simulink model "elec_auto_ev_simulink"  (R2017b)
settings: Solver=FixedStepAuto  StartTime=0.0  StopTime=200  RelTol=1e-3  AbsTol=1e-3
PreLoadFcn:
  | % Simulation parameters
  | dt = 0.01;
  | 
  | % Battery cell parameters
  | ssc_lithium_cell_1RC_ini
  | 
  | % Motor parameters
  | max_torque = 220;
  | max_power = 50e3;
  | 
  | % Vehicle parameters
  | vehicle_mass = 1000;
  | wheel_radius = 0.25;
  | area = 5;
  | drag_coefficient = 0.25;
  | air_density = 1.225;
  | gravity = 9.81;
  | rolling_res_ratio = 0.015;
  | 
  | % Differential drive parameters
  | gear_ratio = 6;
  | 
  | % Simplified braking system parameters
  | force_max_pedal = 500;
  | braking_torque_to_pedal_force_ratio = -4;
  | 
  | % Vehicle controller parameters
  | hill_hold_max_speed = 0.5;
  | 
  | % Water properties for cooling circuit
  | load WaterProperties
undefined symbols (not defined in the file): C1_LUT, Capacity_LUT, cell_Cp_heat, cell_mass, DiscIntNeverNeededParam, Em_LUT, Qe_init, R0_LUT, R1_LUT, sigbuilder_block, SOC_LUT, T_init, Temperature_LUT
libraries: fl_lib x93, nesl_utility x12, LiBatteryElements_lib x4, elec_lib x2, simulink x2, simulink_extras x1
(part 1 of 2)
CloseFcn:
  | try,close(h1_elec_auto_ev),end
  | clear h1_elec_auto_ev
  | try,close(h2_elec_auto_ev),end
  | clear h2_elec_auto_ev
  | 
  | clear simlog_elec_auto_ev
  | clear logsout_elec_auto_ev
Description:
  | Electric Vehicle Configured for HIL
  | 
  | Copyright 2008-2017 The MathWorks, Inc.
settings Model: Creator=MathWorks  LastModifiedBy=Sivakumar
settings SolverCC: InitialStep=1e-3
settings DataIOCC: MaxDataPoints=30000  SaveFormat=Array  SignalLoggingName=logsout_elec_auto_ev
settings OptimizationCC: BlockReduction=off  BooleanDataType=off  LifeSpan=inf
settings DebuggingCC: SaveWithParameterizedLinksMsg=none  UnderspecifiedInitializationDetection=Classic  MergeDetectMultiDrivingBlocksExec=none  SignalResolutionControl=TryResolveAllWithWarning  AllowSymbolicDim=off  SFUnexpectedBacktrackingDiag=warning  SFNoUnconditionalDefaultTransitionDiag=warning  SFExecutionAtInitializationDiag=none
settings HardwareCC: ProdBitPerPointer=32  ProdBitPerSizeT=32  ProdBitPerPtrDiffT=32  ProdLargestAtomicFloat=None  ProdIntDivRoundTo=Undefined  ProdEndianess=Unspecified  ProdWordSize=32  ProdHWDeviceType=32-bit Generic  TargetUnknown=on
settings ModelReferenceCC: PropagateSignalLabelsOutOfModel=off
settings CodeAppCC: StateflowObjectComments=on
settings GRTTargetCC: TargetLangStandard=C89/C90 (ANSI)  GeneratePreprocessorConditionals=Disable all
settings ConfigComp: CovMetricSettings=dw  CovHtmlReporting=on  CovSaveCumulativeToWorkspaceVar=on  CovSaveSingleToWorkspaceVar=on  CovExternalEMLEnable=off  CovSFcnEnable=off
settings SimscapeCC: SimscapeLogType=all  SimscapeLogSimulationStatistics=on  SimscapeLogName=simlog_elec_auto_ev  SimscapeLogDataHistory=30000

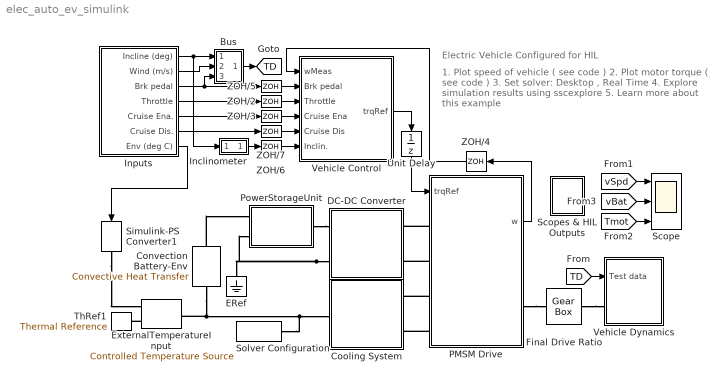
== system elec_auto_ev_simulink ==
  note: Electric Vehicle Configured for HIL
  note: 1. Plot speed of vehicle ( see code )
      | 2. Plot motor torque ( see code )
      | 3. Set solver: Desktop , Real Time
      | 4. Explore simulation results using sscexplore
      | 5. Learn more about this example
  ExternalTemperatureInput : fl_lib/Thermal/Thermal Sources/Controlled Temperature Source
      settings: SourceProductName=Foundation Library
  PowerStorageUnit : Subsystem  mask(Lithium cell (one RC-branch equivalent circuit)){Nseries=50, Nparallel=10, Qe_init=Qe_init, T_init=T_init, Capacity_LUT=Capacity_LUT, Em_LUT=Em_LUT, R0_LUT=R0_LUT, R1_LUT=R1_LUT, C1_LUT=C1_LUT, cell_mass=cell_mass, cell_Cp_heat=cell_Cp_heat, SOC_LUT=SOC_LUT, Temperature_LUT=Temperature_LUT}
      mask prompts: Nseries "Number of series-connected cells"; Nparallel "Number of parallel sets of series-connected cells"; Qe_init "Initial cell charge deficit (A*hr)"; T_init "Initial cell temperature (K)"; Capacity_LUT "Capacity (A*hr, 1xN table)"; Em_LUT "Em open-circuit voltage, Em (volts, MxN table)"; R0_LUT "R0 terminal resistance (ohms, MxN table)"; R1_LUT "R1 cell resistance (ohms, MxN table)"; C1_LUT "C1 capacitance (farads, MxN table)"; cell_mass "Cell mass (kg)"; cell_Cp_heat "Cell specific heat (J/kg/K)"; SOC_LUT "SOC table breakpoints (Mx1 array)"; Temperature_LUT "Temperature table breakpoints (K, 1xN array)"
      mask DialogControl ParameterTabVar0 Prompt: Main
      mask DialogControl ParameterTabVar01 Prompt: Electrical (per cell)
      mask DialogControl ParameterTabVar012 Prompt: Thermal (per cell)
      mask DialogControl ParameterTabVar0123 Prompt: Table Breakpoints
      mask Display:
      | % Battery icon
      | plot([1.8 1.3],[0 0])
      | plot([-0.6 -1.6 -1.6 -2.2],[0 0 -0.9 -0.9])
      | patch([1 1 -1 -1]*0.15+0.7,[-1 1 1 -1]*0.4,[0;0;0]);
      | patch([1 1 -1 -1]*0.15-0.6,[-1 1 1 -1]*0.4,[0;0;0]);
      | patch([1 1 -1 -1]*0.15+1.3,[-1 1 1 -1]*0.8,[0;0;0]);
      | patch([1 1 -1 -1]*0.15-0.0,[-1 1 1 -1]*0.8,[0;0;0]);
      | % Thermal port
      | plot([-1.6,-1.3],[1.2,1.2])
      | plot([-1.6,-1.3],[0.5,0.5])
      | plot([-1.6,-2.5],[0.8,0.8])
      | plot(0.2*sin(0:2*pi/50:2*pi)-1.6,0.35*cos(0:2*pi/50:2*pi)+0.85)
      | plot(0.2*sin(0:2*pi/50:pi)-1.3,0.35*cos(0:2*pi/50:pi)+0.85)
      | 
      | % Plot points to set plot range
      | color('white');plot(2.5,1.5);plot(-2.5,-1.5)
  Bus : Subsystem
  Convection Battery-Env : fl_lib/Thermal/Thermal Elements/Convective Heat Transfer  area=cell_area m^2  heat_tr_coeff=h_conv W/(m^2 * K)  T_specify=off  T_priority=High  T=0 K  T_nominal_specify=off  T_nominal_unit=K  T_nominal_value=1  Q_specify=off  Q_priority=High  Q=0 J/s  Q_nominal_specify=off  Q_nominal_unit=J/s  Q_nominal_value=1
      settings: SourceProductName=Foundation Library
  Cooling System : Subsystem  Tag=PublishSubsystem
  DC-DC Converter : Subsystem
  ERef : fl_lib/Electrical/Electrical Elements/Electrical Reference
      settings: SourceProductName=Foundation Library
  Final Drive Ratio : fl_lib/Mechanical/Mechanisms/Gear Box  ratio=gear_ratio  t_in_specify=off  t_in_priority=High  t_in=0 N*m  t_in_nominal_specify=off  t_in_nominal_unit=N*m  t_in_nominal_value=1  t_out_specify=off  t_out_priority=High  t_out=0 N*m  t_out_nominal_specify=off  t_out_nominal_unit=N*m  t_out_nominal_value=1
      settings: SourceProductName=Foundation Library
  Inclinometer : Subsystem
  Inputs : Subsystem  Tag=STV Subsys  LoadFcn=sigbuilder_block('load');  StartFcn=sigbuilder_block('start');  StopFcn=sigbuilder_block('stop');  ClipboardFcn=sigbuilder_block('clipboard');  mask(Sigbuilder block){tuvar=[0:10]}
      mask help: Simulink:masks:SigbuilderBlock_MD
      mask init:
      | if ~strcmp(get_param(bdroot(gcbh),'SimulationStatus'),'stopped') tuvar = sigbuilder_block('maskInit'); end
      settings: CopyFcn=sigbuilder_block('copy');  DeleteFcn=sigbuilder_block('delete');  ModelCloseFcn=sigbuilder_block('modelClose');  PreSaveFcn=sigbuilder_block('preSave');  PauseFcn=sigbuilder_block('pause');  ContinueFcn=sigbuilder_block('continue');  NameChangeFcn=sigbuilder_block('namechange');  OpenFcn=sigbuilder_block('open',[410.4 81.6 632.4 557.4 ]);  CloseFcn=sigbuilder_block('close');
      mask Display: plot(0, 0, 100, 100,[2, 2, 32, 32, 2], [68, 8, 8, 68, 68],[32, 2], [38, 38], [32, 19, 2],[53, 60, 44], [32, 17, 17, 2],[16, 16, 31, 31]);txt = getActiveGroup(gcbh);text(2, 100, txt,'verticalAlignment', 'top');
  PMSM Drive : Subsystem  Tag=PublishSubsystem  VariantControl=Variant1
  Scope : Scope  NumInputPorts=3
  Scopes & HIL Outputs : Subsystem
  Simulink-PS Converter1 : nesl_utility/Simulink-PS Converter  PhysicalDomain=network_engine_domain  SubClassName=ps_input  LeftPortType=input  RightPortType=output  PseudoPeriodic=off  Frequencies=[]  NoiseDistribution=none  NoiseParameters=[]  Unit=degC  AffineConversion=on  FilteringAndDerivatives=zero  SimscapeFilterOrder=1  InputFilterTimeConstant=.001  UdotUserProvided=1
  Solver Configuration : nesl_utility/Solver Configuration  PhysicalDomain=network_engine_domain  SubClassName=solver  LeftPortType=input  RightPortType=generic  Accelerate=off  Tones=[]  Harmonics=[]  SimulateNoise=off  Profile=off  UseLocalSampling=off  EnableSwitchedLinearOptims=on  FrequencyDomain=off  UseCCode=off  RelTol=0.001  AbsTol=1e-06  MinStep=1e-09  ToWorkspace=off  RevertToSquareIcSolve=off  NumHomotopyIterations=100  PhasorMode=off  PhasorModeNumHarmonics=1  DoDC=off  ResidualTolerance=1e-9  UseLocalSolver=on  LocalSolverChoice=NE_BACKWARD_EULER_ADVANCER  LocalSolverSampleTime=dt  DoFixedCost=on  MaxNonlinIter=3  MaxModeIter=2  LinearAlgebra=Sparse  DelaysMemoryBudget=1024  AutomaticFiltering=on  FilteringTimeConstant=0.001
      settings: AttributesFormatString=Local Solver: %<UseLocalSolver>
  ThRef1 : fl_lib/Thermal/Thermal Elements/Thermal Reference
      settings: SourceProductName=Foundation Library
  Unit Delay : UnitDelay  SampleTime=dt
  Vehicle Dynamics : Subsystem
  Vehicle Control : Subsystem  Tag=PublishSubsystem
  ZOH/{2..7} (6 alike) : ZeroOrderHold  SampleTime=dt
  tag scope: TD=global
  wires:
  Inputs/7(Env (deg C)) -> Simulink-PS Converter1/1
  Inputs/1(Incline (deg)) -> Bus/1(In), Inclinometer/1(a)
  ZOH/2/1 -> Vehicle Control/3(Throttle)
  Inputs/4(Throttle) -> ZOH/2/1
  ZOH/3/1 -> Vehicle Control/4(Cruise Ena)
  Inputs/5(Cruise Ena.) -> ZOH/3/1
  ZOH/5/1 -> Vehicle Control/2(Brk pedal)
  ZOH/6/1 -> Vehicle Control/6(Inclin.)
  ZOH/7/1 -> Vehicle Control/5(Cruise Dis)
  Inputs/3(Brk pedal) -> Bus/3(Br), ZOH/5/1
  ZOH/4/1 -> Vehicle Control/1(wMeas)
  Inputs/6(Cruise Dis.) -> ZOH/7/1
  Inclinometer/1(y) -> ZOH/6/1
  Vehicle Control/1(trqRef) -> Unit Delay/1
  Unit Delay/1 -> PMSM Drive/1(trqRef)
  PMSM Drive/1(w) -> ZOH/4/1
  Inputs/2(Wind (m/s)) -> Bus/2(Wi)
  Bus/1(b) -> [TD]
  [TD] -> Vehicle Dynamics/1(Test data)
  [vSpd] -> Scope/1
  [vBat] -> Scope/2
  [Tmot] -> Scope/3
  connections:
  ExternalTemperatureInput/RConn2 -- ThRef1/LConn1
  Simulink-PS Converter1/RConn1 -- ExternalTemperatureInput/RConn1
  Convection Battery-Env/RConn1 -- PowerStorageUnit/LConn1
  DC-DC Converter/LConn2 -- PowerStorageUnit/LConn2 -- ERef/LConn1
  PowerStorageUnit/RConn1 -- DC-DC Converter/LConn1
  Final Drive Ratio/RConn1 -- Vehicle Dynamics/LConn1
  PMSM Drive/LConn1 -- DC-DC Converter/RConn1
  PMSM Drive/LConn2 -- DC-DC Converter/RConn2
  PMSM Drive/RConn1 -- Final Drive Ratio/LConn1
  Convection Battery-Env/LConn1 -- ExternalTemperatureInput/LConn1 -- Cooling System/LConn1 -- Solver Configuration/RConn1
  PMSM Drive/LConn4 -- Cooling System/RConn2
  PMSM Drive/LConn3 -- Cooling System/RConn1

== system elec_auto_ev_simulink/PowerStorageUnit ==
  note: Scale up voltage drop to total
      | of Ns series-connected cells
  DynamicVoltageInjector : fl_lib/Electrical/Electrical Sources/Controlled Voltage Source
      settings: SourceProductName=Foundation Library
  EnergyInteractionSystem : Subsystem  Tag=PublishSubsystem
  NumCells-1 : fl_lib/Physical Signals/Functions/PS Gain  gain=(Nseries-1)
      settings: SourceProductName=Foundation Library
  Voltage Sensor : fl_lib/Electrical/Electrical Sensors/Voltage Sensor
      settings: SourceProductName=Foundation Library
  + : PMIOPort  Tag=PMCPort  Port=1  Side=Right
  H : PMIOPort  Tag=PMCPort  Port=2  Side=Left
  - : PMIOPort  Tag=PMCPort  Port=3  Side=Left
  connections:
  DynamicVoltageInjector/RConn2 -- -/RConn1
  NumCells-1/RConn1 -- DynamicVoltageInjector/RConn1
  +/RConn1 -- EnergyInteractionSystem/RConn1 -- Voltage Sensor/LConn1
  Voltage Sensor/RConn1 -- NumCells-1/LConn1
  EnergyInteractionSystem/RConn2 -- Voltage Sensor/RConn2 -- DynamicVoltageInjector/LConn1
  H/RConn1 -- EnergyInteractionSystem/LConn1

== system elec_auto_ev_simulink/Bus ==
  In : Inport
  Wi : Inport  Port=2
  Br : Inport  Port=3
  Bus Creator : BusCreator  Inputs=3
  b : Outport
  wires:
  Wi/1 -> Bus Creator/2  "Wind speed"
  Bus Creator/1 -> b/1
  Br/1 -> Bus Creator/3  "Brake pedal"
  In/1 -> Bus Creator/1  "Incline"

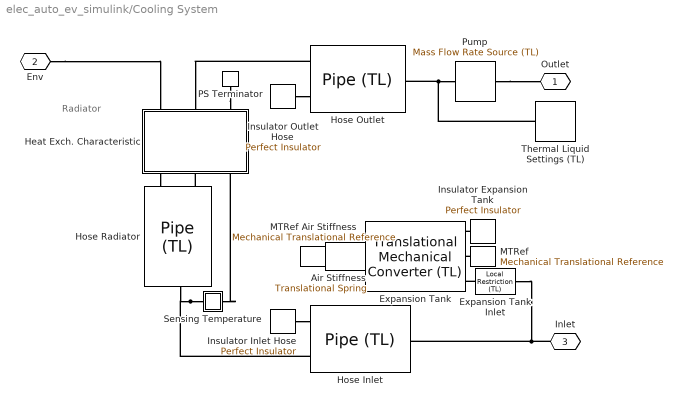
== system elec_auto_ev_simulink/Cooling System ==
  note: Radiator
  Air Stiffness : fl_lib/Mechanical/Translational Elements/Translational Spring  spr_rate=1e3 N/m  v_specify=off  v_priority=High  v=0 m/s  v_nominal_specify=off  v_nominal_unit=m/s  v_nominal_value=1  f_specify=on  f_priority=Low  f=0 N  f_nominal_specify=off  f_nominal_unit=N  f_nominal_value=1  x_specify=off  x_priority=High  x=0 m  x_nominal_specify=off  x_nominal_unit=m  x_nominal_value=1
      settings: SourceProductName=Foundation Library
  Expansion Tank : fl_lib/Thermal Liquid/Elements/Translational Mechanical Converter (TL)  mech_orientation=1  interface_area=pi*50^2 mm^2  x0=200 mm  dead_volume=0.001 m^3  environment_spec=1  environment_pressure=0.101325 MPa  dynamic_compressibility=0  T0=20 degC  p0=1 atm
      settings: SourceProductName=Foundation Library
  Expansion Tank Inlet : fl_lib/Thermal Liquid/Elements/Local Restriction (TL)  restriction_area=pi*10^2 mm^2  area=pi*11^2 mm^2  length=1e-1 m  Cd=0.7  pressure_recovery=0  Re_c=12  mdot_A_specify=off  mdot_A_priority=None  mdot_A=1 kg/s  mdot_A_nominal_specify=off  mdot_A_nominal_unit=kg/s  mdot_A_nominal_value=1
      settings: SourceProductName=Foundation Library
  Heat Exch. Characteristic : Subsystem
  Hose Radiator : fl_lib/Thermal Liquid/Elements/Pipe (TL)  dynamic_compressibility=1  inertia=0  length=2000 mm  area=pi*25^2 mm^2  Dh=50 mm  length_add=500 mm  roughness=1.5e-5 m  Re_lam=2e+3  Re_tur=4e+3  shape_factor=64  Nu_lam=3.66  p0=1 atm  T0=20 degC  mdot0=0.1 kg/s
      settings: SourceProductName=Foundation Library
  Hose Inlet : fl_lib/Thermal Liquid/Elements/Pipe (TL)  dynamic_compressibility=1  inertia=0  length=500 mm  area=pi*25^2 mm^2  Dh=50 mm  length_add=500 mm  roughness=1.5e-5 m  Re_lam=2e+3  Re_tur=4e+3  shape_factor=64  Nu_lam=3.66  p0=1 atm  T0=20 degC  mdot0=0.1 kg/s
      settings: SourceProductName=Foundation Library
  Hose Outlet : fl_lib/Thermal Liquid/Elements/Pipe (TL)  dynamic_compressibility=1  inertia=0  length=500 mm  area=pi*25^2 mm^2  Dh=50 mm  length_add=500 mm  roughness=1.5e-5 m  Re_lam=2e+3  Re_tur=4e+3  shape_factor=64  Nu_lam=3.66  p0=1 atm  T0=20 degC  mdot0=0.1 kg/s
      settings: SourceProductName=Foundation Library
  Insulator Expansion Tank : fl_lib/Thermal/Thermal Elements/Perfect Insulator  T_specify=off  T_priority=High  T=0 K  T_nominal_specify=off  T_nominal_unit=K  T_nominal_value=1
      settings: SourceProductName=Foundation Library
  Insulator Inlet Hose : fl_lib/Thermal/Thermal Elements/Perfect Insulator  T_specify=off  T_priority=High  T=0 K  T_nominal_specify=off  T_nominal_unit=K  T_nominal_value=1
      settings: SourceProductName=Foundation Library
  Insulator Outlet Hose : fl_lib/Thermal/Thermal Elements/Perfect Insulator  T_specify=off  T_priority=High  T=0 K  T_nominal_specify=off  T_nominal_unit=K  T_nominal_value=1
      settings: SourceProductName=Foundation Library
  MTRef : fl_lib/Mechanical/Translational Elements/Mechanical Translational Reference
      settings: SourceProductName=Foundation Library
  MTRef Air Stiffness : fl_lib/Mechanical/Translational Elements/Mechanical Translational Reference
      settings: SourceProductName=Foundation Library
  PS Terminator : fl_lib/Physical Signals/Sinks/PS Terminator
      settings: SourceProductName=Foundation Library
  Pump : fl_lib/Thermal Liquid/Sources/Mass Flow Rate Source (TL)  commanded_mass_flow=0.2 kg/s  area=pi*25^2 mm^2  length=1e-1 m  mdot_A_specify=off  mdot_A_priority=None  mdot_A=1 kg/s  mdot_A_nominal_specify=off  mdot_A_nominal_unit=kg/s  mdot_A_nominal_value=1
      settings: SourceProductName=Foundation Library
  Sensing Temperature : Subsystem
      mask Display: disp('T')
  Thermal Liquid Settings (TL) : fl_lib/Thermal Liquid/Utilities/Thermal Liquid Settings (TL)  table_dimensions=0  T_TLU=T K  p_TLU=p Pa  p_atm=1 atm  pT_region_flag=0  T_min=273.16 K  T_max=373.16 K  p_min=0.1 bar  p_max=500 bar  T_min_1D=273.16 K  T_max_1D=373.16 K  p_min_1D=0.01 MPa  p_max_1D=50 MPa  pT_validity_TLU=ones(11, 12)  rho_parameterization_2D=1  rho_parameterization_1D=1  rho_TLU=rho kg/m^3  beta_TLU=beta Pa  alpha_TLU=alpha 1/K  rho_TLU_2=[999.7973, 999.8431, 1002.3216, 1004.8218, 1007.293, 1009.7358, 1012.1506, 1014.5379, 1016.8979, 1019.2311, 1021.538, 1023.8188; 999.6579, 999.7009, 1002.0303, 1004.382, 1006.7084, 1009.0101, 1011.2874, 1013.5407, 1015.7703, 1017.9766, 1020.1599, 1022.3206; 998.1632, 998.2045, 1000.4375, 1002.6924, 1004.9239, 1007.1324, 1009.3183, 1011.4819, 1013.6236, 1015.7438, 1017.8428, 1019.921; 995.6057, 995.6458, 997.81864, 1000.0128, 1002.1841, 1004.3332, 1006.4603, 1008.566, 1010.6505, 1012.7144, 1014.758, 1016.7815; 992.1724, 992.2119, 994.35133, 996.5113, 998.6484, 1000.7633, 1002.8563, 1004.928, 1006.9788, 1009.009, 1011.0192, 1013.0097; 988.02, 988.0299, 990.15684, 992.3035, 994.4268, 996.5273, 998.6056, 1000.6622, 1002.6976, 1004.7123, 1006.7067, 1008.6813; 983.18, 983.1901, 985.3217, 987.4721, 989.5983, 991.7008, 993.7803, 995.8374, 997.8726, 999.8864, 1001.8795, 1003.8522; 977.75, 977.7583, 979.9094, 982.0783, 984.2216, 986.34, 988.4343, 990.505, 992.5529, 994.5786, 996.5825, 998.5654; 971.77, 971.7836, 973.96734, 976.1678, 978.3409, 980.4876, 982.6087, 984.7049, 986.7768, 988.8254, 990.8511, 992.8545; 965.26, 965.3023, 967.53107, 969.7753, 971.9901, 974.1764, 976.3354, 978.4676, 980.5741, 982.6556, 984.7129, 986.7465; 958.62, 958.6315, 960.627, 962.9267, 965.1944, 967.4314, 969.6387, 971.8173, 973.9681, 976.0921, 978.19, 980.2628] kg/m^3  rho_ref_3=998.21 kg/m^3  T_ref_3=293.16 K  p_ref_3=0.101325 MPa  beta_const_3=2.1791 GPa  alpha_const_3=2.0691e-4 1/K  rho_TLU_4=[999.84; 999.7; 998.2; 995.65; 992.21; 988.03; 983.19; 977.76; 971.78; 965.3; 958.8] kg/m^3  beta_const_4=2.1791 GPa  p_ref_4=0.101325 MPa  rho_ref_5=998.21 kg/m^3  T_ref_5=293.16 K  p_ref_5=0.101325 MPa  beta_const_5=2.1791 GPa  alpha_const_5=2.0691e-4 1/K  u_parameterization_2D=1  u_parameterization_1D=1  u_TLU=u J/g  cp_TLU=Cp J/K/g  u_TLU_2=[.0002, .0018, .086, .1588, .219, .267, .3034, .3288, .3436, .3483, .3435, .3294; 42.062, 42.06, 41.935, 41.804, 41.668, 41.527, 41.382, 41.233, 41.081, 40.924, 40.763, 40.599; 83.953, 83.948, 83.651, 83.349, 83.049, 82.749, 82.451, 82.153, 81.856, 81.56, 81.265, 80.971; 125.77, 125.76, 125.31, 124.86, 124.41, 123.97, 123.53, 123.1, 122.68, 122.25, 121.84, 121.42; 167.57, 167.56, 166.96, 166.37, 165.79, 165.21, 164.65, 164.09, 163.54, 163, 162.46, 161.94; 209.36, 209.36, 208.63, 207.9, 207.19, 206.48, 205.79, 205.11, 204.45, 203.79, 203.14, 202.5; 251.19, 251.19, 250.33, 249.47, 248.62, 247.79, 246.98, 246.18, 245.39, 244.62, 243.86, 243.12; 293.06, 293.06, 292.07, 291.07, 290.1, 289.14, 288.2, 287.28, 286.38, 285.49, 284.62, 283.77; 334.99, 334.99, 333.86, 332.73, 331.63, 330.54, 329.48, 328.44, 327.41, 326.41, 325.43, 324.46; 377, 377, 375.73, 374.46, 373.22, 372, 370.81, 369.64, 368.5, 367.38, 366.27, 365.19; 419.01, 419.01, 417.69, 416.27, 414.89, 413.54, 412.21, 410.91, 409.64, 408.4, 407.17, 405.98] kJ/kg  cp_TLU_3=[4.2199, 4.2194, 4.1957, 4.1726, 4.1508, 4.13, 4.1103, 4.0916, 4.0738, 4.0569, 4.0408, 4.0254; 4.1955, 4.1951, 4.1769, 4.1592, 4.1422, 4.1259, 4.1103, 4.0954, 4.0812, 4.0676, 4.0545, 4.0421; 4.1843, 4.184, 4.169, 4.1543, 4.1401, 4.1264, 4.1133, 4.1007, 4.0885, 4.0768, 4.0656, 4.0548; 4.1801, 4.1798, 4.1667, 4.1538, 4.1413, 4.1293, 4.1177, 4.1064, 4.0956, 4.0851, 4.075, 4.0653; 4.1796, 4.1794, 4.1675, 4.1558, 4.1444, 4.1334, 4.1227, 4.1123, 4.1023, 4.0926, 4.0832, 4.0741; 4.1813, 4.1813, 4.1702, 4.1592, 4.1484, 4.138, 4.1279, 4.1181, 4.1086, 4.0993, 4.0903, 4.0816; 4.185, 4.185, 4.1742, 4.1636, 4.1532, 4.1432, 4.1334, 4.1239, 4.1146, 4.1056, 4.0969, 4.0884; 4.1901, 4.1901, 4.1795, 4.169, 4.1588, 4.1489, 4.1393, 4.1299, 4.1207, 4.1118, 4.1032, 4.0947; 4.1968, 4.1968, 4.1862, 4.1757, 4.1655, 4.1555, 4.1458, 4.1364, 4.1273, 4.1183, 4.1096, 4.1012; 4.2052, 4.2052, 4.1944, 4.1837, 4.1733, 4.1632, 4.1534, 4.1438, 4.1345, 4.1255, 4.1166, 4.108; 4.2136, 4.2136, 4.2045, 4.1935, 4.1828, 4.1724, 4.1623, 4.1524, 4.1429, 4.1335, 4.1245, 4.1157] kJ/kg/K  u_TLU_4=[.0018; 42.06; 83.948; 125.76; 167.56; 209.36; 251.19; 293.06; 334.99; 377; 418.01] kJ/kg  cp_TLU_5=[4.2199; 4.1955; 4.1843; 4.1801; 4.1796; 4.1813; 4.185; 4.1901; 4.1968; 4.2052; 4.2136] kJ/kg/K  nu_TLU=nu cm^2/s  nu_TLU_2=[1.7917; 1.3061; 1.0032; .8006; .6577; .553; .4739; .4127; .3643; .3254; .2866] mm^2/s  k_TLU=k mW/m/K  k_TLU_2=[561.04; 580.02; 598.44; 615.48; 630.6; 643.61; 654.39; 663.13; 670.02; 675.27; 680.52] mW/m/K
      settings: SourceProductName=Foundation Library
  Outlet : PMIOPort  Port=1  Side=Right
  Env : PMIOPort  Port=2  Side=Left
  Inlet : PMIOPort  Port=3  Side=Right
  connections:
  Insulator Outlet Hose/LConn1 -- Hose Outlet/LConn2
  Insulator Inlet Hose/LConn1 -- Hose Inlet/LConn2
  Env/RConn1 -- Heat Exch. Characteristic/RConn1
  Thermal Liquid Settings (TL)/RConn1 -- Hose Outlet/RConn1 -- Pump/LConn1
  Hose Outlet/LConn1 -- Heat Exch. Characteristic/RConn2
  Pump/RConn1 -- Outlet/RConn1
  Inlet/RConn1 -- Expansion Tank Inlet/LConn1 -- Hose Inlet/RConn1
  Sensing Temperature/LConn1 -- Hose Radiator/RConn1 -- Hose Inlet/LConn1
  Hose Radiator/LConn1 -- Heat Exch. Characteristic/LConn2
  Heat Exch. Characteristic/LConn1 -- Hose Radiator/LConn2
  Sensing Temperature/RConn1 -- Heat Exch. Characteristic/LConn3
  PS Terminator/LConn1 -- Heat Exch. Characteristic/RConn3
  Insulator Expansion Tank/LConn1 -- Expansion Tank/LConn3
  Air Stiffness/RConn1 -- MTRef Air Stiffness/LConn1
  Air Stiffness/LConn1 -- Expansion Tank/RConn1
  Expansion Tank Inlet/RConn1 -- Expansion Tank/LConn1
  MTRef/LConn1 -- Expansion Tank/LConn2

== system elec_auto_ev_simulink/DC-DC Converter ==
  DC-DC Converter : elec_lib/Sources/DC-DC Converter  v_ref=400 V  P_rated=60 kW  droop_param=2  droop=0.1 V/A  droop_percent=1  reversible=1  efficiency=98  P_fixed=100 W  model_dynamics=0  tau=0.02 s  v_ini=400 V  i1_max=1000 A  fault_condition=1  fault_threshold=0.5
      settings: SourceProductName=Simscape Electronics  SourceProductBaseCode=SN
  No faults : fl_lib/Physical Signals/Sources/PS Constant  constant=0
      settings: SourceProductName=Foundation Library
  Resistor : fl_lib/Electrical/Electrical Elements/Resistor  R=0.002 Ohm  i_specify=off  i_priority=None  i=0 A  i_nominal_specify=off  i_nominal_unit=A  i_nominal_value=1  v_specify=off  v_priority=None  v=0 V  v_nominal_specify=off  v_nominal_unit=V  v_nominal_value=1
      settings: SourceProductName=Foundation Library
  Sensing Battery Quantities : Subsystem
  Vbat+ : PMIOPort  Port=1  Side=Left
  V+ : PMIOPort  Tag=PMCPort  Port=2  Side=Right
  Vbat- : PMIOPort  Port=3  Side=Left
  V- : PMIOPort  Tag=PMCPort  Port=4  Side=Right
  connections:
  No faults/RConn1 -- DC-DC Converter/LConn3
  DC-DC Converter/RConn2 -- V-/RConn1 -- DC-DC Converter/LConn2 -- Vbat-/RConn1 -- Sensing Battery Quantities/LConn1
  Vbat+/RConn1 -- Sensing Battery Quantities/RConn1
  Sensing Battery Quantities/RConn2 -- DC-DC Converter/LConn1
  DC-DC Converter/RConn1 -- Resistor/LConn1
  Resistor/RConn1 -- V+/RConn1

== system elec_auto_ev_simulink/Inclinometer ==
  a : Inport
  Trigonometric Function : Trigonometry
  d2r : Gain  Gain=pi/180
  g : Gain  Gain=gravity
  y : Outport
  wires:
  Trigonometric Function/1 -> g/1
  a/1 -> d2r/1
  d2r/1 -> Trigonometric Function/1
  g/1 -> y/1

== system elec_auto_ev_simulink/Inputs ==
  Demux : Demux  Tag=STV Demux  Outputs=7
  FromWs : FromWorkspace  Tag=STV FromWs  VariableName=tuvar  SampleTime=0.01
      SigBuilderData=|
      | common.afterFinalStr = 'Extrapolate'
      | common.sampleTime = '0.01'
      | dataSet.timeRange = [0 200]
      | dataSet.name = 'Test 1'
      | sbobj.Name = 'Signal Builder'
      | sbobj.Groups.Name = 'Test 1'
      | sbobj.Groups.Signals(1).Name = 'Incline (deg)'
      | sbobj.Groups.Signals(1).XData = [0 100 100 200]
      | sbobj.Groups.Signals(1).YData = [10 10 -10 -10]
      | sbobj.Groups.Signals(2).Name = 'Wind (m/s)'
      | sbobj.Groups.Signals(2).XData = [0 200]
      | sbobj.Groups.Signals(2).YData = [0 0]
      | sbobj.Groups.Signals(3).Name = 'Brk pedal'
      | sbobj.Groups.Signals(3).XData = [0 180 180 200]
      | sbobj.Groups.Signals(3).YData = [0 0 1 1]
      | sbobj.Groups.Signals(4).Name = 'Throttle'
      | sbobj.Groups.Signals(4).XData = [0 0.1 0.3 7.5 7.7 200]
      | sbobj.Groups.Signals(4).YData = [0 0 1 1 0 0]
      | sbobj.Groups.Signals(5).Name = 'Cruise Ena.'
      | sbobj.Groups.Signals(5).XData = [0 8 8 10 10 200]
      | sbobj.Groups.Signals(5).YData = [0 0 1 1 0 0]
      | sbobj.Groups.Signals(6).Name = 'Cruise Dis.'
      | sbobj.Groups.Signals(6).XData = [0 200]
      | sbobj.Groups.Signals(6).YData = [0 0]
      | sbobj.Groups.Signals(7).Name = 'Env (deg C)'
      | sbobj.Groups.Signals(7).XData = [0 200]
      | sbobj.Groups.Signals(7).YData = [25 25]
      | sbobj.Groups.TimeRange = [0 200]
  Incline (deg) : Outport  Tag=STV Outport
  Wind (m/s) : Outport  Tag=STV Outport  Port=2
  Brk pedal : Outport  Tag=STV Outport  Port=3
  Throttle : Outport  Tag=STV Outport  Port=4
  Cruise Ena. : Outport  Tag=STV Outport  Port=5
  Cruise Dis. : Outport  Tag=STV Outport  Port=6
  Env (deg C) : Outport  Tag=STV Outport  Port=7
  wires:
  FromWs/1 -> Demux/1
  Demux/1 -> Incline (deg)/1
  Demux/2 -> Wind (m/s)/1
  Demux/3 -> Brk pedal/1
  Demux/4 -> Throttle/1
  Demux/5 -> Cruise Ena./1
  Demux/6 -> Cruise Dis./1
  Demux/7 -> Env (deg C)/1

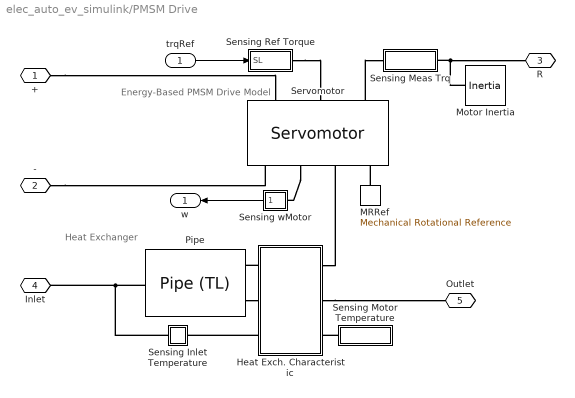
== system elec_auto_ev_simulink/PMSM Drive ==
  note: Energy-Based
      | PMSM Drive Model
  note: Heat Exchanger
  trqRef : Inport
  Heat Exch. Characteristic : Subsystem
  MRRef : fl_lib/Mechanical/Rotational Elements/Mechanical Rotational Reference
      settings: SourceProductName=Foundation Library
  Motor Inertia : fl_lib/Mechanical/Rotational Elements/Inertia  inertia=0.02 kg*m^2  w_specify=on  w_priority=High  w=0 rpm  w_nominal_specify=off  w_nominal_unit=rad/s  w_nominal_value=1  t_specify=off  t_priority=High  t=0 N*m  t_nominal_specify=off  t_nominal_unit=N*m  t_nominal_value=1
      settings: SourceProductName=Foundation Library
  Pipe : fl_lib/Thermal Liquid/Elements/Pipe (TL)  dynamic_compressibility=1  inertia=0  length=400 mm  area=pi*25^2 mm^2  Dh=50 mm  length_add=500 mm  roughness=1.5e-5 m  Re_lam=2e+3  Re_tur=4e+3  shape_factor=64  Nu_lam=3.66  p0=1 atm  T0=20 degC  mdot0=0.1 kg/s
      settings: SourceProductName=Foundation Library
  Sensing Inlet Temperature : Subsystem
      mask Display: disp('T');
  Sensing Meas Trq : Subsystem
      mask Display: disp('trqMeas')
  Sensing Motor Temperature : Subsystem
      mask Display: disp('Tmotor')
  Sensing Ref Torque : Subsystem
      mask Display: disp('trqRef')
  Sensing wMotor : Subsystem
      mask Display: disp('w');
  Servomotor : elec_lib/Actuators & Drivers/Rotational Actuators/Servomotor  torque_speed_param=2  w_t=[ 0 3.75e+3 7.5e+3 8e+3 ] rpm  T_t=[max_torque max_torque max_torque 0] N*m  torque_max=max_torque N*m  power_max=max_power W  Tc=0.02 s  losses_param=1  eff=96  w_eff=1500 rpm  T_eff=50 N*m  Piron=200 W  Pbase=0 W  w_eff_vec=[-8000 -4000 0 4000 8000] rpm  T_eff_vec=[0 0.03 0.06 0.09] N*m  losses_mat=[1.49 1.67 2.21 3.10; 0.42 0.69 1.14 2.03; 0.06 0.24 0.78 1.68; 0.42 0.69 1.14 2.03; 1.49 1.67 2.21 3.10] W  efficiency_mat=[95 95 95 95; 95 95 95 95; 95 95 95 95; 95 95 95 95; 95 95 95 95]  Res=0 Ohm  J=0 kg*m^2  lam=1e-5 N*m/(rad/s)  speed0=0 rpm  faulted_specify=off  faulted_priority=None  faulted=0  faulted_nominal_specify=off  faulted_nominal_unit=1  faulted_nominal_value=1  alpha=0.00393 1/K  Tmeas=25 degC  Tmeas2=125 degC  losses_mat_T2=[1.49 1.74 2.49 3.74;0.42 0.67 1.42 2.67;0.06 0.31 1.06 2.31;0.42 0.67 1.42 2.67;1.49 1.74 2.49 3.74] W  efficiency_mat_T2=[95 95 95 95; 95 95 95 95; 95 95 95 95; 95 95 95 95; 95 95 95 95]  thermal_mass=1500 J/K  initial_temperature=20 degC  fault_condition=1  fault_threshold=0.5
      settings: SourceProductName=Simscape Electronics  SourceProductBaseCode=SN
  + : PMIOPort  Port=1  Side=Left
  - : PMIOPort  Port=2  Side=Left
  R : PMIOPort  Port=3  Side=Right
  Inlet : PMIOPort  Port=4  Side=Left
  Outlet : PMIOPort  Port=5  Side=Left
  w : Outport
  wires:
  trqRef/1 -> Sensing Ref Torque/1(SL)
  Sensing wMotor/1(SL) -> w/1
  connections:
  -/RConn1 -- Servomotor/RConn1
  +/RConn1 -- Servomotor/LConn1
  Pipe/RConn1 -- Sensing Inlet Temperature/LConn1 -- Inlet/RConn1
  Heat Exch. Characteristic/RConn2 -- Outlet/RConn1
  Heat Exch. Characteristic/RConn1 -- Servomotor/RConn3
  Servomotor/LConn3 -- Sensing Meas Trq/LConn1
  MRRef/LConn1 -- Servomotor/RConn4
  Motor Inertia/LConn1 -- R/RConn1 -- Sensing Meas Trq/RConn1
  Sensing Ref Torque/RConn1 -- Servomotor/LConn2
  Servomotor/RConn2 -- Sensing wMotor/LConn1
  Sensing Motor Temperature/LConn1 -- Heat Exch. Characteristic/RConn3
  Heat Exch. Characteristic/LConn3 -- Sensing Inlet Temperature/RConn1
  Heat Exch. Characteristic/LConn1 -- Pipe/LConn2
  Pipe/LConn1 -- Heat Exch. Characteristic/LConn2

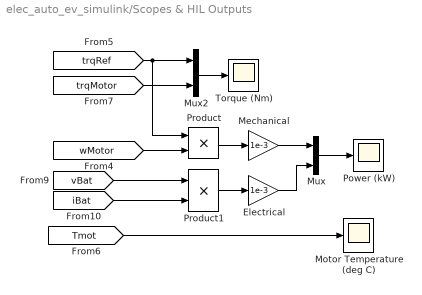
== system elec_auto_ev_simulink/Scopes & HIL Outputs ==
  " Electrical " : Gain  Gain=1e-3
  Mechanical : Gain  Gain=1e-3
  Motor Temperature (deg C) : Scope
  Mux : Mux  Inputs=2
  Mux2 : Mux  Inputs=2
  Power (kW) : Scope
  Product : Product
  Product1 : Product
  Torque (Nm) : Scope
  wires:
  [wMotor] -> Product/2
  [trqRef] -> Mux2/1, Product/1
  Product/1 -> Mechanical/1
  [Tmot] -> Motor Temperature (deg C)/1
  [trqMotor] -> Mux2/2
  [vBat] -> Product1/1
  [iBat] -> Product1/2
  Product1/1 -> " Electrical "/1
  Mechanical/1 -> Mux/1
  " Electrical "/1 -> Mux/2
  Mux/1 -> Power (kW)/1
  Mux2/1 -> Torque (Nm)/1

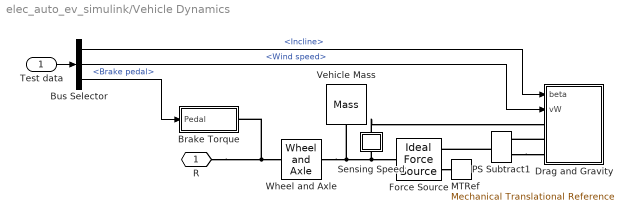
== system elec_auto_ev_simulink/Vehicle Dynamics ==
  Test data : Inport
  Brake Torque : Subsystem
  Bus Selector : BusSelector  OutputSignals=Incline,Wind speed,Brake pedal
  Drag and Gravity : Subsystem
  Force Source : fl_lib/Mechanical/Mechanical Sources/Ideal Force Source
      settings: SourceProductName=Foundation Library
  MTRef : fl_lib/Mechanical/Translational Elements/Mechanical Translational Reference
      settings: SourceProductName=Foundation Library
  PS Subtract1 : fl_lib/Physical Signals/Functions/PS Subtract
      settings: SourceProductName=Foundation Library
  Sensing Speed : Subsystem
      mask Display: disp('v')
  Vehicle Mass : fl_lib/Mechanical/Translational Elements/Mass  mass=vehicle_mass kg  v_specify=off  v_priority=High  v=0 m/s  v_nominal_specify=off  v_nominal_unit=m/s  v_nominal_value=1  f_specify=off  f_priority=High  f=0 N  f_nominal_specify=off  f_nominal_unit=N  f_nominal_value=1
      settings: SourceProductName=Foundation Library
  Wheel and Axle : fl_lib/Mechanical/Mechanisms/Wheel and Axle  R=wheel_radius m  or=1  t_specify=off  t_priority=High  t=0 N*m  t_nominal_specify=off  t_nominal_unit=N*m  t_nominal_value=1  f_specify=off  f_priority=High  f=0 N  f_nominal_specify=off  f_nominal_unit=N  f_nominal_value=1
      settings: SourceProductName=Foundation Library
  R : PMIOPort  Port=1  Side=Left
  wires:
  Test data/1 -> Bus Selector/1
  Bus Selector/3 -> Brake Torque/1(Pedal)  "<Brake pedal>"
  Bus Selector/1 -> Drag and Gravity/1(beta)  "<Incline>"
  Bus Selector/2 -> Drag and Gravity/2(vW)  "<Wind speed>"
  connections:
  Force Source/RConn2 -- MTRef/LConn1
  R/RConn1 -- Brake Torque/RConn1 -- Wheel and Axle/LConn1
  PS Subtract1/RConn1 -- Force Source/RConn1
  PS Subtract1/LConn1 -- Drag and Gravity/LConn3
  Drag and Gravity/LConn2 -- PS Subtract1/LConn2
  Wheel and Axle/RConn1 -- Sensing Speed/LConn1 -- Force Source/LConn1 -- Vehicle Mass/LConn1
  Sensing Speed/RConn1 -- Drag and Gravity/LConn1

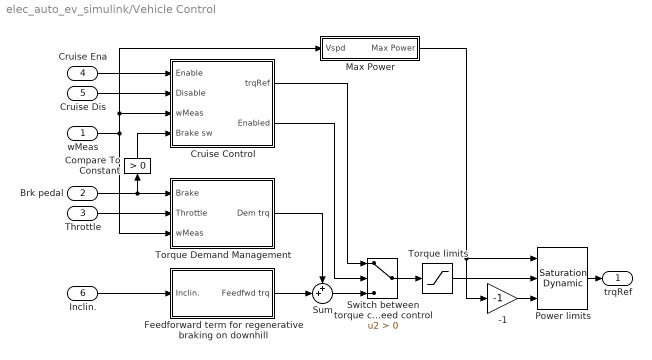
== system elec_auto_ev_simulink/Vehicle Control ==
  wMeas : Inport
  Brk pedal : Inport  Port=2
  Throttle : Inport  Port=3
  Cruise Ena : Inport  Port=4
  Cruise Dis : Inport  Port=5
  Inclin. : Inport  Port=6
  -1 : Gain  Gain=-1
  Compare To Constant : simulink/Logic and Bit Operations/Compare To Constant  relop=>  const=0  OutDataTypeStr=boolean
  Cruise Control : Subsystem
  Feedforward term for regenerative braking on downhill : Subsystem
  Max Power : Subsystem
  Power limits : simulink/Discontinuities/Saturation Dynamic  OutMin=[]  OutMax=[]  OutDataTypeStr=Inherit: Same as second input  OutDataType=fixdt(1, 16)  OutScaling=2^-10  DoSatur=off
  Sum : Sum  Inputs=++|
  Switch between torque control and speed control : Switch  Criteria=u2 > Threshold
  Torque limits : Saturate  UpperLimit=max_torque  LowerLimit=-max_torque
  Torque Demand Management : Subsystem
  trqRef : Outport
  wires:
  Switch between torque control and speed control/1 -> Torque limits/1
  Cruise Ena/1 -> Cruise Control/1(Enable)
  wMeas/1 -> Max Power/1(Vspd), Cruise Control/3(wMeas), Torque Demand Management/3(wMeas)
  Cruise Control/1(trqRef) -> Switch between torque control and speed control/1
  Cruise Control/2(Enabled) -> Switch between torque control and speed control/2
  Cruise Dis/1 -> Cruise Control/2(Disable)
  Compare To Constant/1 -> Cruise Control/4(Brake sw)
  Throttle/1 -> Torque Demand Management/2(Throttle)
  Brk pedal/1 -> Torque Demand Management/1(Brake), Compare To Constant/1
  Inclin./1 -> Feedforward term for regenerative braking on downhill/1(Inclin.)
  Torque Demand Management/1(Dem trq) -> Sum/1
  Sum/1 -> Switch between torque control and speed control/3
  Feedforward term for regenerative braking on downhill/1(Feedfwd trq) -> Sum/2
  Torque limits/1 -> Power limits/2
  Power limits/1 -> trqRef/1
  -1/1 -> Power limits/3
  Max Power/1(Max Power) -> -1/1, Power limits/1

== system elec_auto_ev_simulink/PowerStorageUnit/EnergyInteractionSystem ==
  note: Equivalent Circuit Model for Single Battery Cell
  CapDynamicElement : LiBatteryElements_lib/C_table  C_Table=C1_LUT*Nparallel F  SOC_Table=SOC_LUT  Temp_Table=Temperature_LUT K  v0=0 V
  Em_table : LiBatteryElements_lib/Em_table  C_Table=Capacity_LUT*Nparallel hr*A  Em_Table=Em_LUT V  SOC_Table=SOC_LUT  Temp_Table=Temperature_LUT K  Qinit=Qe_init*Nparallel hr*A
  NumCells : fl_lib/Physical Signals/Functions/PS Gain  gain=Nseries
      settings: SourceProductName=Foundation Library
  Power Sum : fl_lib/Physical Signals/Functions/PS Add
      settings: SourceProductName=Foundation Library
  ResInternalA : LiBatteryElements_lib/R_table  R_Table=R0_LUT/Nparallel Ohm  SOC_Table=SOC_LUT  Temp_Table=Temperature_LUT K
  ResInternalB : LiBatteryElements_lib/R_table  R_Table=R1_LUT/Nparallel Ohm  SOC_Table=SOC_LUT  Temp_Table=Temperature_LUT K
  HeatManagementBlock : Subsystem
  + : PMIOPort  Port=1  Side=Right
  - : PMIOPort  Port=2  Side=Right
  H : PMIOPort  Tag=PMCPort  Port=3  Side=Left
  connections:
  NumCells/LConn1 -- Power Sum/RConn1
  +/RConn1 -- ResInternalA/RConn1
  CapDynamicElement/LConn2 -- HeatManagementBlock/RConn1 -- Em_table/RConn2 -- ResInternalA/LConn2 -- ResInternalB/LConn2
  Em_table/LConn1 -- ResInternalB/LConn1 -- CapDynamicElement/LConn1
  ResInternalB/RConn2 -- Power Sum/LConn2
  ResInternalA/RConn2 -- Power Sum/LConn1
  CapDynamicElement/RConn1 -- ResInternalB/RConn1 -- ResInternalA/LConn1
  Em_table/RConn1 -- -/RConn1
  ResInternalA/LConn3 -- Em_table/LConn3 -- CapDynamicElement/LConn3 -- ResInternalB/LConn3
  NumCells/RConn1 -- HeatManagementBlock/LConn1
  H/RConn1 -- HeatManagementBlock/LConn2

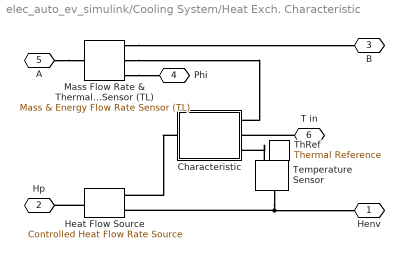
== system elec_auto_ev_simulink/Cooling System/Heat Exch. Characteristic ==
  Characteristic : Subsystem
  Heat Flow Source : fl_lib/Thermal/Thermal Sources/Controlled Heat Flow Rate Source
      settings: SourceProductName=Foundation Library
  Mass Flow Rate & Thermal Flux Sensor (TL) : fl_lib/Thermal Liquid/Sensors/Mass & Energy Flow Rate Sensor (TL)
      settings: SourceProductName=Foundation Library
  Temperature Sensor : fl_lib/Thermal/Thermal Sensors/Temperature Sensor
      settings: SourceProductName=Foundation Library
  ThRef : fl_lib/Thermal/Thermal Elements/Thermal Reference
      settings: SourceProductName=Foundation Library
  Henv : PMIOPort  Port=1  Side=Right
  Hp : PMIOPort  Port=2  Side=Left
  B : PMIOPort  Port=3  Side=Right
  Phi : PMIOPort  Port=4  Side=Right
  A : PMIOPort  Port=5  Side=Left
  T in : PMIOPort  Port=6  Side=Left
  connections:
  A/RConn1 -- Mass Flow Rate & Thermal Flux Sensor (TL)/LConn1
  Temperature Sensor/LConn1 -- Henv/RConn1 -- Heat Flow Source/RConn2
  ThRef/LConn1 -- Temperature Sensor/RConn1
  Heat Flow Source/LConn1 -- Hp/RConn1
  Mass Flow Rate & Thermal Flux Sensor (TL)/RConn1 -- B/RConn1
  Mass Flow Rate & Thermal Flux Sensor (TL)/RConn3 -- Phi/RConn1
  Mass Flow Rate & Thermal Flux Sensor (TL)/RConn2 -- Characteristic/RConn1
  T in/RConn1 -- Characteristic/RConn2
  Temperature Sensor/RConn2 -- Characteristic/RConn3
  Characteristic/LConn1 -- Heat Flow Source/RConn1

== system elec_auto_ev_simulink/Cooling System/Sensing Temperature ==
  Pressure & Temperature Sensor (TL) : fl_lib/Thermal Liquid/Sensors/Pressure & Temperature Sensor (TL)
      settings: SourceProductName=Foundation Library
  TLRef : fl_lib/Thermal Liquid/Elements/Absolute Reference (TL)
      settings: SourceProductName=Foundation Library
  T : PMIOPort  Port=1  Side=Right
  A : PMIOPort  Port=2  Side=Left
  connections:
  Pressure & Temperature Sensor (TL)/RConn3 -- T/RConn1
  TLRef/LConn1 -- Pressure & Temperature Sensor (TL)/RConn1
  A/RConn1 -- Pressure & Temperature Sensor (TL)/LConn1

== system elec_auto_ev_simulink/DC-DC Converter/Sensing Battery Quantities ==
  Battery Voltage : nesl_utility/PS-Simulink Converter  PhysicalDomain=network_engine_domain  SubClassName=ps_output  LeftPortType=input  RightPortType=output  PseudoPeriodic=off  Frequencies=[]  Unit=V  AffineConversion=off
  Current Sensor : fl_lib/Electrical/Electrical Sensors/Current Sensor
      settings: SourceProductName=Foundation Library
  PS-Simulink Converter1 : nesl_utility/PS-Simulink Converter  PhysicalDomain=network_engine_domain  SubClassName=ps_output  LeftPortType=input  RightPortType=output  PseudoPeriodic=off  Frequencies=[]  Unit=A  AffineConversion=off
  Voltage Sensor : fl_lib/Electrical/Electrical Sensors/Voltage Sensor
      settings: SourceProductName=Foundation Library
  +1 : PMIOPort  Port=1  Side=Right
  - : PMIOPort  Port=2  Side=Left
  +2 : PMIOPort  Port=3  Side=Right
  tag scope: iBat=global, vBat=global
  wires:
  Battery Voltage/1 -> [vBat]
  PS-Simulink Converter1/1 -> [iBat]
  connections:
  Voltage Sensor/RConn2 -- -/RConn1
  Voltage Sensor/LConn1 -- Current Sensor/LConn1 -- +1/RConn1
  Voltage Sensor/RConn1 -- Battery Voltage/LConn1
  Current Sensor/RConn2 -- +2/RConn1
  Current Sensor/RConn1 -- PS-Simulink Converter1/LConn1

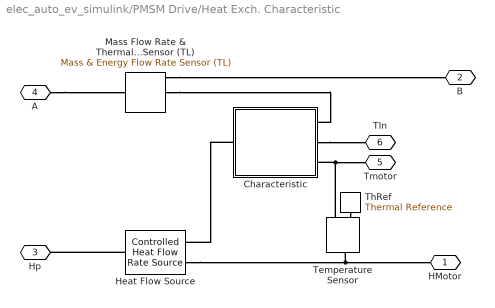
== system elec_auto_ev_simulink/PMSM Drive/Heat Exch. Characteristic ==
  Characteristic : Subsystem
  Heat Flow Source : fl_lib/Thermal/Thermal Sources/Controlled Heat Flow Rate Source
      settings: SourceProductName=Foundation Library
  Mass Flow Rate & Thermal Flux Sensor (TL) : fl_lib/Thermal Liquid/Sensors/Mass & Energy Flow Rate Sensor (TL)
      settings: SourceProductName=Foundation Library
  Temperature Sensor : fl_lib/Thermal/Thermal Sensors/Temperature Sensor
      settings: SourceProductName=Foundation Library
  ThRef : fl_lib/Thermal/Thermal Elements/Thermal Reference
      settings: SourceProductName=Foundation Library
  HMotor : PMIOPort  Port=1  Side=Right
  B : PMIOPort  Port=2  Side=Right
  Hp : PMIOPort  Port=3  Side=Left
  A : PMIOPort  Port=4  Side=Left
  Tmotor : PMIOPort  Port=5  Side=Right
  TIn : PMIOPort  Port=6  Side=Left
  connections:
  Mass Flow Rate & Thermal Flux Sensor (TL)/RConn1 -- B/RConn1
  Heat Flow Source/RConn2 -- HMotor/RConn1 -- Temperature Sensor/LConn1
  ThRef/LConn1 -- Temperature Sensor/RConn1
  Heat Flow Source/LConn1 -- Hp/RConn1
  A/RConn1 -- Mass Flow Rate & Thermal Flux Sensor (TL)/LConn1
  Temperature Sensor/RConn2 -- Tmotor/RConn1 -- Characteristic/LConn3
  Mass Flow Rate & Thermal Flux Sensor (TL)/RConn2 -- Characteristic/LConn1
  Characteristic/LConn2 -- TIn/RConn1
  Characteristic/RConn1 -- Heat Flow Source/RConn1

== system elec_auto_ev_simulink/PMSM Drive/Sensing Inlet Temperature ==
  Pressure & Temperature Sensor (TL) : fl_lib/Thermal Liquid/Sensors/Pressure & Temperature Sensor (TL)
      settings: SourceProductName=Foundation Library
  TLRef : fl_lib/Thermal Liquid/Elements/Absolute Reference (TL)
      settings: SourceProductName=Foundation Library
  A : PMIOPort  Port=1  Side=Left
  T : PMIOPort  Port=2  Side=Right
  connections:
  Pressure & Temperature Sensor (TL)/RConn3 -- T/RConn1
  Pressure & Temperature Sensor (TL)/LConn1 -- A/RConn1
  TLRef/LConn1 -- Pressure & Temperature Sensor (TL)/RConn1

== system elec_auto_ev_simulink/PMSM Drive/Sensing Meas Trq ==
  Ideal Torque Sensor : fl_lib/Mechanical/Mechanical Sensors/Ideal Torque Sensor
      settings: SourceProductName=Foundation Library
  PS-Simulink Converter2 : nesl_utility/PS-Simulink Converter  PhysicalDomain=network_engine_domain  SubClassName=ps_output  LeftPortType=input  RightPortType=output  PseudoPeriodic=off  Frequencies=[]  Unit=N*m  AffineConversion=off
  R : PMIOPort  Port=1  Side=Left
  C : PMIOPort  Port=2  Side=Right
  tag scope: trqMotor=global
  wires:
  PS-Simulink Converter2/1 -> [trqMotor]
  connections:
  C/RConn1 -- Ideal Torque Sensor/RConn1
  R/RConn1 -- Ideal Torque Sensor/LConn1
  Ideal Torque Sensor/RConn2 -- PS-Simulink Converter2/LConn1

== system elec_auto_ev_simulink/PMSM Drive/Sensing Motor Temperature ==
  Motor Temperature : nesl_utility/PS-Simulink Converter  PhysicalDomain=network_engine_domain  SubClassName=ps_output  LeftPortType=input  RightPortType=output  PseudoPeriodic=off  Frequencies=[]  Unit=degC  AffineConversion=on
  PS : PMIOPort  Port=1  Side=Left
  tag scope: Tmot=global
  wires:
  Motor Temperature/1 -> [Tmot]
  connections:
  Motor Temperature/LConn1 -- PS/RConn1

== system elec_auto_ev_simulink/PMSM Drive/Sensing Ref Torque ==
  SL : Inport
  Simulink-PS G1 : nesl_utility/Simulink-PS Converter  PhysicalDomain=network_engine_domain  SubClassName=ps_input  LeftPortType=input  RightPortType=output  PseudoPeriodic=off  Frequencies=[]  NoiseDistribution=none  NoiseParameters=[]  Unit=1  AffineConversion=off  FilteringAndDerivatives=zero  SimscapeFilterOrder=1  InputFilterTimeConstant=1e-6  UdotUserProvided=1
  PS : PMIOPort  Port=1  Side=Right
  tag scope: trqRef=global
  wires:
  SL/1 -> Simulink-PS G1/1, [trqRef]
  connections:
  Simulink-PS G1/RConn1 -- PS/RConn1

== system elec_auto_ev_simulink/PMSM Drive/Sensing wMotor ==
  PS-Simulink Converter : nesl_utility/PS-Simulink Converter  PhysicalDomain=network_engine_domain  SubClassName=ps_output  LeftPortType=input  RightPortType=output  PseudoPeriodic=off  Frequencies=[]  Unit=rad/s  AffineConversion=off
  PS : PMIOPort  Port=1  Side=Left
  SL : Outport
  tag scope: wMotor=global
  wires:
  PS-Simulink Converter/1 -> SL/1, [wMotor]
  connections:
  PS/RConn1 -- PS-Simulink Converter/LConn1

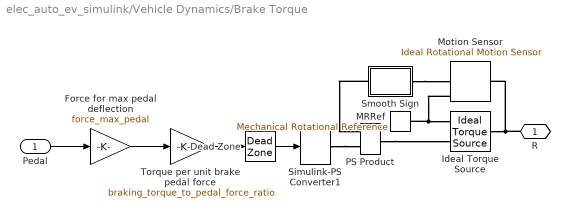
== system elec_auto_ev_simulink/Vehicle Dynamics/Brake Torque ==
  Pedal : Inport
  Dead Zone : DeadZone  LowerValue=-max_torque*gear_ratio  UpperValue=max_torque*gear_ratio  SaturateOnIntegerOverflow=on
  Force for max pedal deflection : Gain  Gain=force_max_pedal
  Ideal Torque Source : fl_lib/Mechanical/Mechanical Sources/Ideal Torque Source
      settings: SourceProductName=Foundation Library
  MRRef : fl_lib/Mechanical/Rotational Elements/Mechanical Rotational Reference
      settings: SourceProductName=Foundation Library
  Motion Sensor : fl_lib/Mechanical/Mechanical Sensors/Ideal Rotational Motion Sensor  offset=0 rad
      settings: SourceProductName=Foundation Library
  PS Product : fl_lib/Physical Signals/Functions/PS Product
      settings: SourceProductName=Foundation Library
  Simulink-PS Converter1 : nesl_utility/Simulink-PS Converter  PhysicalDomain=network_engine_domain  SubClassName=ps_input  LeftPortType=input  RightPortType=output  PseudoPeriodic=off  Frequencies=[]  NoiseDistribution=none  NoiseParameters=[]  Unit=N*m  AffineConversion=off  FilteringAndDerivatives=zero  SimscapeFilterOrder=1  InputFilterTimeConstant=0.001  UdotUserProvided=1
  Smooth Sign : Subsystem
  Torque per unit brake pedal force : Gain  Gain=braking_torque_to_pedal_force_ratio
  R : PMIOPort  Port=1  Side=Right
  wires:
  Pedal/1 -> Force for max pedal deflection/1
  Force for max pedal deflection/1 -> Torque per unit brake pedal force/1
  Torque per unit brake pedal force/1 -> Dead Zone/1
  Dead Zone/1 -> Simulink-PS Converter1/1
  connections:
  Smooth Sign/RConn1 -- PS Product/LConn2
  Motion Sensor/RConn1 -- MRRef/LConn1 -- Ideal Torque Source/RConn2
  Ideal Torque Source/LConn1 -- Motion Sensor/LConn1 -- R/RConn1
  PS Product/RConn1 -- Ideal Torque Source/RConn1
  Simulink-PS Converter1/RConn1 -- PS Product/LConn1
  Smooth Sign/LConn1 -- Motion Sensor/RConn2

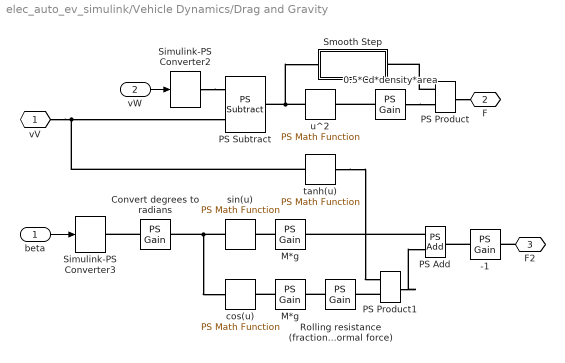
== system elec_auto_ev_simulink/Vehicle Dynamics/Drag and Gravity ==
  beta : Inport
  vW : Inport  Port=2
  " M*g " : fl_lib/Physical Signals/Functions/PS Gain  gain=vehicle_mass*gravity
      settings: SourceProductName=Foundation Library
  -1 : fl_lib/Physical Signals/Functions/PS Gain  gain=-1
      settings: SourceProductName=Foundation Library
  0.5*Cd*density*area : fl_lib/Physical Signals/Functions/PS Gain  gain=0.5*drag_coefficient*air_density*area
      settings: SourceProductName=Foundation Library
  "Convert degrees to radians " : fl_lib/Physical Signals/Functions/PS Gain  gain=pi/180
      settings: SourceProductName=Foundation Library
  M*g : fl_lib/Physical Signals/Functions/PS Gain  gain=vehicle_mass*gravity
      settings: SourceProductName=Foundation Library
  PS Add : fl_lib/Physical Signals/Functions/PS Add
      settings: SourceProductName=Foundation Library
  PS Product : fl_lib/Physical Signals/Functions/PS Product
      settings: SourceProductName=Foundation Library
  PS Product1 : fl_lib/Physical Signals/Functions/PS Product
      settings: SourceProductName=Foundation Library
  PS Subtract : fl_lib/Physical Signals/Functions/PS Subtract
      settings: SourceProductName=Foundation Library
  "Rolling resistance (fraction of normal force) " : fl_lib/Physical Signals/Functions/PS Gain  gain=rolling_res_ratio
      settings: SourceProductName=Foundation Library
  Simulink-PS Converter2 : nesl_utility/Simulink-PS Converter  PhysicalDomain=network_engine_domain  SubClassName=ps_input  LeftPortType=input  RightPortType=output  PseudoPeriodic=off  Frequencies=[]  NoiseDistribution=none  NoiseParameters=[]  Unit=N*m  AffineConversion=off  FilteringAndDerivatives=zero  SimscapeFilterOrder=1  InputFilterTimeConstant=0.001  UdotUserProvided=1
  Simulink-PS Converter3 : nesl_utility/Simulink-PS Converter  PhysicalDomain=network_engine_domain  SubClassName=ps_input  LeftPortType=input  RightPortType=output  PseudoPeriodic=off  Frequencies=[]  NoiseDistribution=none  NoiseParameters=[]  Unit=N*m  AffineConversion=off  FilteringAndDerivatives=zero  SimscapeFilterOrder=1  InputFilterTimeConstant=0.001  UdotUserProvided=1
  Smooth Step : Subsystem
  cos(u) : fl_lib/Physical Signals/Functions/PS Math Function  fcn_choice=2
      settings: SourceProductName=Foundation Library
  sin(u) : fl_lib/Physical Signals/Functions/PS Math Function  fcn_choice=1
      settings: SourceProductName=Foundation Library
  tanh(u) : fl_lib/Physical Signals/Functions/PS Math Function  fcn_choice=10
      settings: SourceProductName=Foundation Library
  u^2 : fl_lib/Physical Signals/Functions/PS Math Function  fcn_choice=7
      settings: SourceProductName=Foundation Library
  vV : PMIOPort  Port=1  Side=Left
  F : PMIOPort  Port=2  Side=Left
  F2 : PMIOPort  Port=3  Side=Left
  wires:
  vW/1 -> Simulink-PS Converter2/1
  beta/1 -> Simulink-PS Converter3/1
  connections:
  vV/RConn1 -- tanh(u)/LConn1 -- PS Subtract/LConn1
  Simulink-PS Converter2/RConn1 -- PS Subtract/LConn2
  u^2/LConn1 -- Smooth Step/LConn1 -- PS Subtract/RConn1
  0.5*Cd*density*area/LConn1 -- u^2/RConn1
  0.5*Cd*density*area/RConn1 -- PS Product/LConn2
  PS Product/RConn1 -- F/RConn1
  PS Product/LConn1 -- Smooth Step/RConn1
  "Convert degrees to radians "/LConn1 -- Simulink-PS Converter3/RConn1
  sin(u)/LConn1 -- "Convert degrees to radians "/RConn1 -- cos(u)/LConn1
  M*g/LConn1 -- sin(u)/RConn1
  " M*g "/LConn1 -- cos(u)/RConn1
  "Rolling resistance (fraction of normal force) "/LConn1 -- " M*g "/RConn1
  PS Product1/LConn2 -- "Rolling resistance (fraction of normal force) "/RConn1
  PS Add/LConn1 -- M*g/RConn1
  PS Product1/RConn1 -- PS Add/LConn2
  -1/LConn1 -- PS Add/RConn1
  F2/RConn1 -- -1/RConn1
  tanh(u)/RConn1 -- PS Product1/LConn1

== system elec_auto_ev_simulink/Vehicle Dynamics/Sensing Speed ==
  MTRef : fl_lib/Mechanical/Translational Elements/Mechanical Translational Reference
      settings: SourceProductName=Foundation Library
  Motion Sensor : fl_lib/Mechanical/Mechanical Sensors/Ideal Translational Motion Sensor  offset=0 m
      settings: SourceProductName=Foundation Library
  PS-Simulink Converter3 : nesl_utility/PS-Simulink Converter  PhysicalDomain=network_engine_domain  SubClassName=ps_output  LeftPortType=input  RightPortType=output  PseudoPeriodic=off  Frequencies=[]  Unit=mph  AffineConversion=off
  R : PMIOPort  Port=1  Side=Left
  w : PMIOPort  Port=2  Side=Right
  tag scope: vSpd=global
  wires:
  PS-Simulink Converter3/1 -> [vSpd]  "Vehicle Speed"
  connections:
  R/RConn1 -- Motion Sensor/LConn1
  MTRef/LConn1 -- Motion Sensor/RConn1
  Motion Sensor/RConn2 -- PS-Simulink Converter3/LConn1 -- w/RConn1

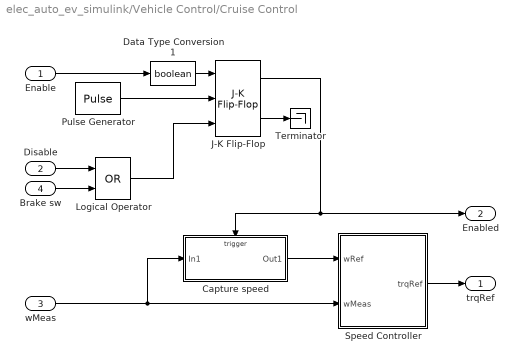
== system elec_auto_ev_simulink/Vehicle Control/Cruise Control ==
  Enable : Inport
  Disable : Inport  Port=2
  wMeas : Inport  Port=3
  Brake sw : Inport  Port=4
  Capture speed : Subsystem  TreatAsAtomicUnit=on
  Data Type Conversion1 : DataTypeConversion  OutDataTypeStr=boolean
  J-K Flip-Flop : simulink_extras/Flip Flops/J-K Flip-Flop  initial_condition=0
      settings: SourceProductName=Simulink Extras
  Logical Operator : Logic  Operator=OR  AllPortsSameDT=off  OutDataTypeStr=boolean
  Pulse Generator : DiscretePulseGenerator  Period=10  PulseWidth=5  SampleTime=0.01
  Speed Controller : Subsystem  mask(P+I motor speed controller){Kp=100, Ki=100, trqMax=max_torque, ts=dt}
      mask prompts: Kp "Proportional gain (Nm/(rad/s))"; Ki "Integral gain (Nm/rad)"; trqMax "Maximum torque demand"; ts "Sample time"
      mask help: Inputs wRef and wMeas are the demanded rotor speed and measured rotor speed in rad/s. The controller output is a torque demand in Nm.
  Terminator : Terminator
  trqRef : Outport
  Enabled : Outport  Port=2
  wires:
  Enable/1 -> Data Type Conversion1/1
  Pulse Generator/1 -> J-K Flip-Flop/2
  Disable/1 -> Logical Operator/1
  Speed Controller/1(trqRef) -> trqRef/1
  Brake sw/1 -> Logical Operator/2
  wMeas/1 -> Capture speed/1(In1), Speed Controller/2(wMeas)
  Logical Operator/1 -> J-K Flip-Flop/3
  J-K Flip-Flop/1 -> Enabled/1, Capture speed/Trigger
  Data Type Conversion1/1 -> J-K Flip-Flop/1
  J-K Flip-Flop/2 -> Terminator/1
  Capture speed/1(Out1) -> Speed Controller/1(wRef)

== system elec_auto_ev_simulink/Vehicle Control/Feedforward term for regenerative braking on downhill ==
  Inclin. : Inport
  " M " : Gain  Gain=vehicle_mass
  1/ratio : Gain  Gain=1/gear_ratio
  Wheel radius : Gain  Gain=wheel_radius
  Feedfwd trq : Outport
  wires:
  Inclin./1 -> " M "/1
  " M "/1 -> Wheel radius/1
  Wheel radius/1 -> 1/ratio/1  "Wheel torque"
  1/ratio/1 -> Feedfwd trq/1  "Motor torque"
